simulink model "SMC_Reaching_Law"  (R2025a)
settings: Solver=FixedStepAuto  StartTime=0.0  StopTime=10.0  FixedStep=0.001  RelTol=1e-3
settings Model: Creator=1  LastModifiedBy=1

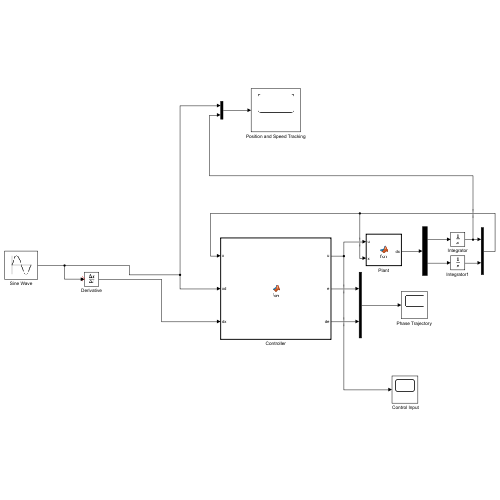
[thumbnail: Simulink's stored preview of the top-level diagram]
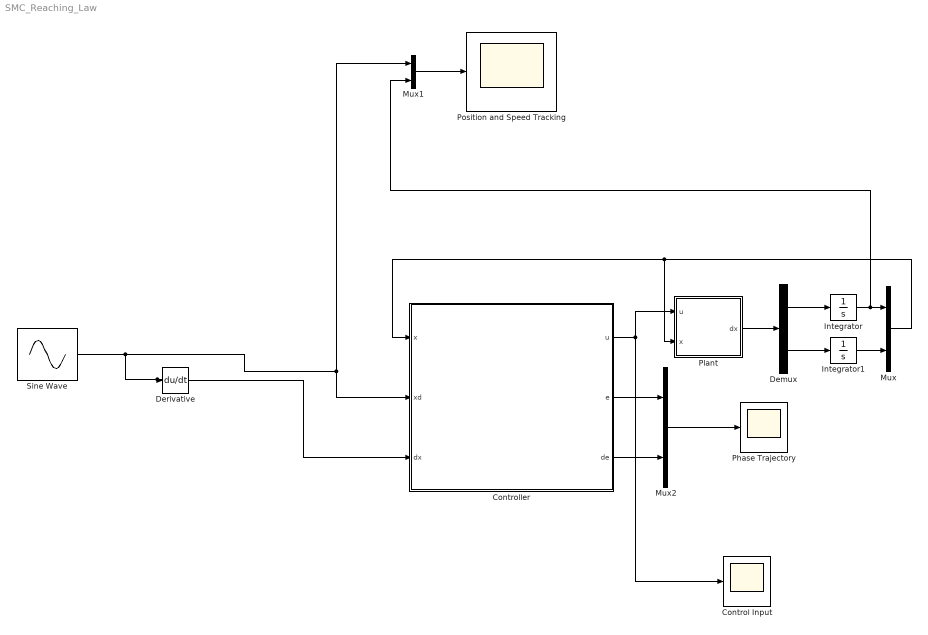
== system SMC_Reaching_Law ==
  " Control Input" : Scope
      settings: ActiveDisplayYMinimum=-0.3  ActiveDisplayYMaximum=0.5  DataLoggingVariableName=ScopeData2
  Controller : MATLAB Function  TreatAsAtomicUnit=on
  Demux : Demux  Outputs=2
  Derivative : Derivative
  Integrator : Integrator  InitialCondition=-0.15
  Integrator1 : Integrator  InitialCondition=0.15
  Mux : Mux  Inputs=2
  Mux1 : Mux  Inputs=2
  Mux2 : Mux  Inputs=2
  Phase Trajectory : Scope
      settings: ActiveDisplayYMinimum=-1.2534902620200516  ActiveDisplayYMaximum=1.4538671860946959
  Plant : MATLAB Function  TreatAsAtomicUnit=on
  Position and Speed Tracking : Scope
      settings: ActiveDisplayYMinimum=-2.0000000000000004  ActiveDisplayYMaximum=4.0000000000000018
  Sine Wave : Sin  SampleTime=0
  wires:
  Controller/1(u) -> " Control Input"/1, Plant/1(u)
  Plant/1(dx) -> Demux/1
  Demux/1 -> Integrator/1
  Demux/2 -> Integrator1/1
  Derivative/1 -> Controller/3(dx)
  Controller/2(e) -> Mux2/1
  Controller/3(de) -> Mux2/2
  Mux2/1 -> Phase Trajectory/1
  Integrator1/1 -> Mux/2
  Sine Wave/1 -> Mux1/1, Controller/2(xd), Derivative/1
  Mux1/1 -> Position and Speed Tracking/1
  Mux/1 -> Plant/2(x), Controller/1(x)
  Integrator/1 -> Mux1/2, Mux/1

== matlab function SMC_Reaching_Law/Plant ==
  data: u input; x input; dx output
function dx = fcn(u, x)
% Plant dynamics based on the paper:
% dx1 = x2
% dx2 = -25*x2 + 133*u + d(t)

% 입력:
% x: 현재 상태 벡터 [x1; x2] → 위치, 속도
% u: 제어 입력 (controller output)

% 외란 설정
d = 10.1;

% 상태 미분 계산
dx = zeros(2,1);
dx(1) = x(2);                      % x1_dot = x2
dx(2) = -25 * x(2) + 133 * u + d;  % x2_dot = 모델 + 외란

== matlab function SMC_Reaching_Law/Controller ==
  data: x input; u output; xd input; dx input; e output; de output
function [u, e, de] = fcn(x, xd, dx)
% x   : 현재 상태 [x1; x2]
% xd  : 기준 위치
% dx  : 기준 속도

% 파라미터 설정
c = 15;
k = 10;
N = 0.5;
b = 133;

% 모델링된 시스템의 비선형 항
f = -25 * x(2);

% 오차 계산
e  = xd - x(1);
de = dx - x(2);

% 슬라이딩 함수
s = c * e + de;

% 제어 입력
u = (1 / b) * (c * e + de - f + N * sign(s) + k * s);
